simulink model "HubDepotModel"  (Simulink 7.9)
settings: Solver=VariableStepDiscrete  StartTime=0.0  StopTime=100.0  RelTol=1e-3
undefined symbols (not defined in the file or in its folder): CustomerBase_1
libraries: simeventslib x10
(part 4 of 4)

== matlab function Depot_3/Storage_Subsystem/<<SOURCE>> Source_Stocked_Product/Schedule_Product_Deliveries_CONTROL/Reorder_Control ==
  data: Inventory_Position input double; Reorder_Point input double; Reorder_Quantity input double; Component input double; out_Inventory_Position output double; out_Reorder_Signal output double; out_Reorder_Quantity output double
function [out_Inventory_Position, out_Reorder_Signal, out_Reorder_Quantity] = fcn(Inventory_Position, Reorder_Point, Reorder_Quantity, Component)
%This function is a combination of all the CONTROL systems at once

out_Inventory_Position = Inventory_Position;
out_Reorder_Signal =0;
out_Reorder_Quantity = 0;
if eq(Component, 0) == 0
    %Operative Subsystem Control
    if Inventory_Position(Component) <= Reorder_Point(Component)
        out_Reorder_Signal = Reorder_Quantity(Component);
        out_Reorder_Quantity = Reorder_Quantity(Component);
        
        %Control & Monitoring Subsystem
        out_Inventory_Position(Component) = Inventory_Position(Component) + Reorder_Quantity(Component);
        
    end
end

== matlab function Depot_3/Storage_Subsystem/<<SOURCE>> Source_Stocked_Product/Transfer_Product_CONTROL/Calculate_Inventory ==
  data: Net_Inventory input double; out_Inventory output double; Component input double; Shipment_Quantity input double
function out_Inventory = fcn(Net_Inventory, Component, Shipment_Quantity)
%#codegen

%coder.extrinsic('str2num');

%y = zeros(1, 'int32');
%y = Type;
out_Inventory = Net_Inventory;
if eq(Component, 0) == 0
    out_Inventory(Component) = Net_Inventory(Component) + Shipment_Quantity;
end

end

== matlab function Depot_4/Storage_Subsystem/<<DELIVER>>Deliver_Stocked_Product/Deliver_Stocked_Product_CONTROL/Calculate_Inventory_C ==
  data: Net_Inventory input double; Inventory_Position input double; out_Net_Inventory output double; Component input double; Consumption_Quantity input double; out_Inventory_Position output double
function [out_Net_Inventory,out_Inventory_Position] = fcn(Net_Inventory, Inventory_Position, Component, Consumption_Quantity)
%#codegen

%coder.extrinsic('str2num');

%y = zeros(1, 'int32');
%y = Type;
out_Net_Inventory = Net_Inventory;
out_Inventory_Position = Inventory_Position;
if eq(Component, 0) == 0
    out_Net_Inventory(Component) = Net_Inventory(Component) - Consumption_Quantity;
    out_Inventory_Position(Component) = Inventory_Position(Component) - Consumption_Quantity;
end

end

== matlab function Depot_4/Storage_Subsystem/<<SOURCE>> Source_Stocked_Product/Schedule_Product_Deliveries_CONTROL/Reorder_Control ==
  data: Inventory_Position input double; Reorder_Point input double; Reorder_Quantity input double; Component input double; out_Inventory_Position output double; out_Reorder_Signal output double; out_Reorder_Quantity output double
function [out_Inventory_Position, out_Reorder_Signal, out_Reorder_Quantity] = fcn(Inventory_Position, Reorder_Point, Reorder_Quantity, Component)
%This function is a combination of all the CONTROL systems at once

out_Inventory_Position = Inventory_Position;
out_Reorder_Signal =0;
out_Reorder_Quantity = 0;
if eq(Component, 0) == 0
    %Operative Subsystem Control
    if Inventory_Position(Component) <= Reorder_Point(Component)
        out_Reorder_Signal = Reorder_Quantity(Component);
        out_Reorder_Quantity = Reorder_Quantity(Component);
        
        %Control & Monitoring Subsystem
        out_Inventory_Position(Component) = Inventory_Position(Component) + Reorder_Quantity(Component);
        
    end
end

== matlab function Depot_4/Storage_Subsystem/<<SOURCE>> Source_Stocked_Product/Transfer_Product_CONTROL/Calculate_Inventory ==
  data: Net_Inventory input double; out_Inventory output double; Component input double; Shipment_Quantity input double
function out_Inventory = fcn(Net_Inventory, Component, Shipment_Quantity)
%#codegen

%coder.extrinsic('str2num');

%y = zeros(1, 'int32');
%y = Type;
out_Inventory = Net_Inventory;
if eq(Component, 0) == 0
    out_Inventory(Component) = Net_Inventory(Component) + Shipment_Quantity;
end

end
